simulink model "idex2_hzc_2017b"  (R2017b)
settings: Solver=ode4  StartTime=0.0  StopTime=400.0  FixedStep=0.1  MaxStep=0.01  RelTol=1e-8
libraries: simulink_extras x5, simulink x1
settings Model: Creator=erange  LastModifiedBy=erange
settings DataIOCC: LimitDataPoints=on  SaveFormat=Array  SignalLoggingSaveFormat=ModelDataLogs  SignalLoggingName=sigsOut
settings OptimizationCC: InitFltsAndDblsToZero=on  LifeSpan=inf
settings DebuggingCC: SaveWithParameterizedLinksMsg=none  UnderspecifiedInitializationDetection=Classic  MergeDetectMultiDrivingBlocksExec=none  SignalResolutionControl=TryResolveAllWithWarning  MultiTaskDSMMsg=warning  MultiTaskCondExecSysMsg=none  FcnCallInpInsideContextMsg=warning  SFUnexpectedBacktrackingDiag=warning  SFNoUnconditionalDefaultTransitionDiag=warning  SFExecutionAtInitializationDiag=none
settings HardwareCC: ProdBitPerPointer=32  ProdBitPerSizeT=32  ProdBitPerPtrDiffT=32  ProdLargestAtomicFloat=None  ProdIntDivRoundTo=Undefined  ProdEndianess=Unspecified  ProdWordSize=32  ProdHWDeviceType=32-bit Generic  TargetUnknown=on
settings ModelReferenceCC: PropagateSignalLabelsOutOfModel=off
settings SFSimCC: SimUseLocalCustomCode=on
settings RTWCC: Description=Generic Real-Time Target  RTWUseLocalCustomCode=on
settings CodeAppCC: StateflowObjectComments=on
settings GRTTargetCC: TargetFcnLib=ansi_tfl_tmw.mat  TargetLangStandard=C89/C90 (ANSI)  CombineOutputUpdateFcns=off  GRTInterface=on
settings ConfigComp: CovMetricSettings=dw  CovHtmlReporting=on  CovSaveCumulativeToWorkspaceVar=on  CovSaveSingleToWorkspaceVar=on

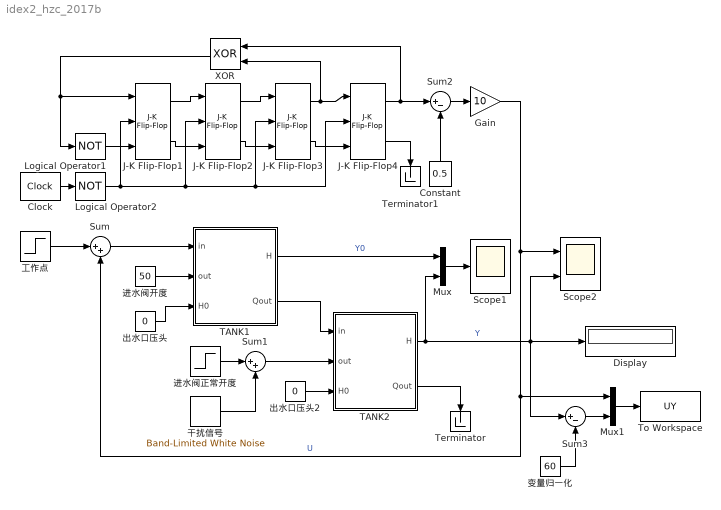
== system idex2_hzc_2017b ==
  Clock : simulink_extras/Flip Flops/Clock  period=2
  Constant : Constant  Value=0.5
  Display : Display
  Gain : Gain  Gain=10  SaturateOnIntegerOverflow=on  OutDataTypeStr=Inherit: Same as input  ParamDataTypeStr=Inherit: Same as input
  J-K Flip-Flop{1..4} (4 alike) : simulink_extras/Flip Flops/J-K Flip-Flop  initial_condition=1
      settings: SourceProductName=Simulink
  Logical Operator1 : Logic  Operator=NOT  Inputs=1  AllPortsSameDT=off
  Logical Operator2 : Logic  Operator=NOT  Inputs=1  AllPortsSameDT=off
  Mux : Mux  Inputs=2
  Mux1 : Mux  Inputs=2
  Scope1 : Scope
  Scope2 : Scope  NumInputPorts=2
  Sum : Sum  Inputs=|++  SaturateOnIntegerOverflow=on
  Sum1 : Sum  Inputs=|++  SaturateOnIntegerOverflow=on
  Sum2 : Sum  Inputs=|+-  SaturateOnIntegerOverflow=on
  Sum3 : Sum  Inputs=|+-  SaturateOnIntegerOverflow=on
  TANK1 : Subsystem  mask(TANK){A=500, Kin=350, Kout=50, Ts=2}
      mask prompts: Ts "sample time"
      mask help:
      | Adh/dt=Kin*u1-Kout*u2*Sqrt(h-u3)
      |     y1=h
      |     y2=Qout
      mask Display:
      | plot([0,0,10,10,0],[0,10,10,0,0],[0,10],[7,7],[2,8],[6,6],[4,6],[5,5]);
      | port_label('output', 1, 'H ');
      | port_label('output', 2, 'Qo ');
      | port_label('input', 1, ' U1');
      | port_label('input', 2, ' U2');
      | port_label('input', 3, ' Ho');
  TANK2 : Subsystem  mask(TANK){A=400, Kin=1, Kout=45, Ts=2}
      mask prompts: Ts "Sample time"
      mask help:
      | Adh/dt=Kin*u1-Kout*u2*Sqrt(h-u3)
      |     y1=h
      |     y2=Qout
      mask Display:
      | plot([0,0,10,10,0],[0,10,10,0,0],[0,10],[7,7],[2,8],[6,6],[4,6],[5,5]);
      | port_label('output', 1, 'H ');
      | port_label('output', 2, 'Qo ');
      | port_label('input', 1, ' U1');
      | port_label('input', 2, ' U2');
      | port_label('input', 3, ' Ho');
  Terminator : Terminator
  Terminator1 : Terminator
  To Workspace : ToWorkspace  VariableName=UY  SampleTime=2
  XOR : Logic  Operator=XOR  AllPortsSameDT=off
  出水口压头 : Constant  Value=0
  出水口压头2 : Constant  Value=0
  变量归一化 : Constant  Value=60
  工作点 : Step  Time=0  After=50  SampleTime=2
  干扰信号 : simulink/Sources/Band-Limited White Noise  Cov=0  Ts=2  seed=[23341]
  "进水阀开度 " : Constant  Value=50
  进水阀正常开度 : Step  Time=0  After=50  SampleTime=2
  wires:
  工作点/1 -> Sum/1
  Sum/1 -> TANK1/1(in)
  TANK1/2(Qout) -> TANK2/1(in)
  "进水阀开度 "/1 -> TANK1/2(out)
  Sum1/1 -> TANK2/2(out)
  进水阀正常开度/1 -> Sum1/1
  干扰信号/1 -> Sum1/2
  出水口压头2/1 -> TANK2/3(H0)
  TANK2/2(Qout) -> Terminator/1
  TANK2/1(H) -> Mux/2, Scope2/2, Sum3/1, Display/1  "Y"
  Mux/1 -> Scope1/1
  TANK1/1(H) -> Mux/1  "Y0"
  出水口压头/1 -> TANK1/3(H0)
  J-K Flip-Flop1/1 -> J-K Flip-Flop2/1
  J-K Flip-Flop4/1 -> XOR/1, Sum2/1
  XOR/1 -> J-K Flip-Flop1/1, Logical Operator1/1
  J-K Flip-Flop3/2 -> J-K Flip-Flop4/3
  J-K Flip-Flop1/2 -> J-K Flip-Flop2/3
  Logical Operator1/1 -> J-K Flip-Flop1/3
  J-K Flip-Flop3/1 -> J-K Flip-Flop4/1, XOR/2
  J-K Flip-Flop4/2 -> Terminator1/1
  Sum2/1 -> Gain/1
  Constant/1 -> Sum2/2
  J-K Flip-Flop2/2 -> J-K Flip-Flop3/3
  J-K Flip-Flop2/1 -> J-K Flip-Flop3/1
  Clock/1 -> Logical Operator2/1
  Logical Operator2/1 -> J-K Flip-Flop4/2, J-K Flip-Flop3/2, J-K Flip-Flop2/2, J-K Flip-Flop1/2
  Gain/1 -> Sum/2, Mux1/1, Scope2/1  "U"
  Mux1/1 -> To Workspace/1
  Sum3/1 -> Mux1/2
  变量归一化/1 -> Sum3/2

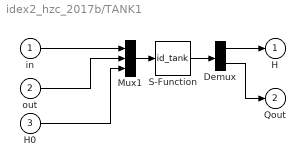
== system idex2_hzc_2017b/TANK1 ==
  in : Inport
  out : Inport  Port=2
  H0 : Inport  Port=3
  Demux : Demux  Outputs=2
  Mux1 : Mux  Inputs=3
  S-Function : S-Function  FunctionName=id_tank  Parameters=A, Kin,Kout,Ts  SFunctionDeploymentMode=off  EnableBusSupport=off
  H : Outport
  Qout : Outport  Port=2
  wires:
  H0/1 -> Mux1/3
  Demux/2 -> Qout/1
  Demux/1 -> H/1
  S-Function/1 -> Demux/1
  in/1 -> Mux1/1
  out/1 -> Mux1/2
  Mux1/1 -> S-Function/1

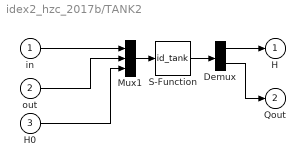
== system idex2_hzc_2017b/TANK2 ==
  in : Inport
  out : Inport  Port=2
  H0 : Inport  Port=3
  Demux : Demux  Outputs=2
  Mux1 : Mux  Inputs=3
  S-Function : S-Function  FunctionName=id_tank  Parameters=A, Kin,Kout, Ts  SFunctionDeploymentMode=off  EnableBusSupport=off
  H : Outport
  Qout : Outport  Port=2
  wires:
  Mux1/1 -> S-Function/1
  out/1 -> Mux1/2
  in/1 -> Mux1/1
  S-Function/1 -> Demux/1
  Demux/1 -> H/1
  Demux/2 -> Qout/1
  H0/1 -> Mux1/3
